simulink model "data_inspector_Baleka"  (R2024a)
settings: Solver=ode45  StartTime=0.0  StopTime=Sim.time  MaxStep=0.00001  RelTol=1e-12  AbsTol=1e-12
settings Model: Creator=heath  LastModifiedBy=Gavin

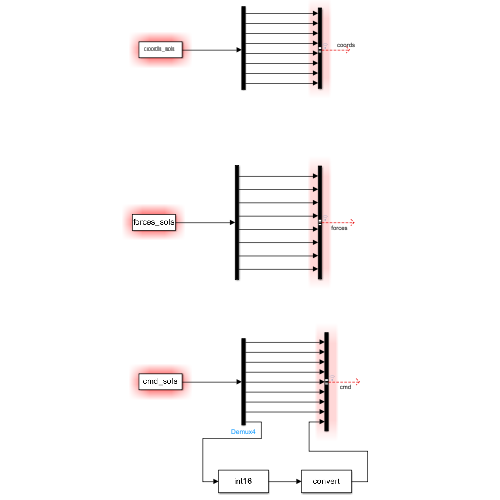
[thumbnail: Simulink's stored preview of the top-level diagram]
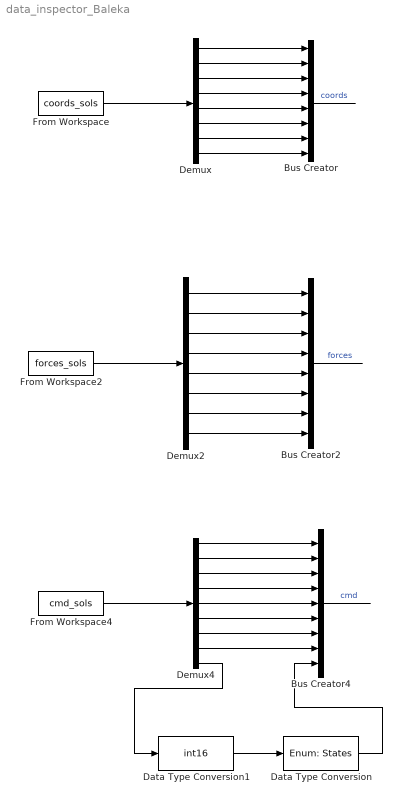
== system data_inspector_Baleka ==
  Bus Creator : BusCreator  Inputs=8  OutDataTypeStr=Bus: Coordinate
      settings: InheritFromInputs=off
  Bus Creator2 : BusCreator  Inputs=8  OutDataTypeStr=Bus: Forces
      settings: InheritFromInputs=off
  Bus Creator4 : BusCreator  Inputs=9  OutDataTypeStr=Bus: Cmd
      settings: InheritFromInputs=off
  Data Type Conversion : DataTypeConversion  OutDataTypeStr=Enum: States  SaturateOnIntegerOverflow=off  RndMeth=Floor
  Data Type Conversion1 : DataTypeConversion  OutDataTypeStr=int16  SaturateOnIntegerOverflow=off  RndMeth=Floor
  Demux : Demux  Outputs=8
  Demux2 : Demux  Outputs=8
  Demux4 : Demux  Outputs=9
  From Workspace : FromWorkspace  VariableName=coords_sols
  From Workspace2 : FromWorkspace  VariableName=forces_sols
  From Workspace4 : FromWorkspace  VariableName=cmd_sols
  wires:
  From Workspace2/1 -> Demux2/1
  Bus Creator/1 -> ?  "coords"
  Demux/8 -> Bus Creator/8
  Demux/7 -> Bus Creator/7
  Demux/6 -> Bus Creator/6
  Demux/5 -> Bus Creator/5
  Demux/4 -> Bus Creator/4
  Demux/3 -> Bus Creator/3
  Demux/2 -> Bus Creator/2
  Demux/1 -> Bus Creator/1
  From Workspace/1 -> Demux/1
  Bus Creator2/1 -> ?  "forces"
  From Workspace4/1 -> Demux4/1
  Demux4/2 -> Bus Creator4/2
  Demux4/1 -> Bus Creator4/1
  Demux4/5 -> Bus Creator4/5
  Demux4/3 -> Bus Creator4/3
  Demux4/4 -> Bus Creator4/4
  Bus Creator4/1 -> ?  "cmd"
  Demux2/6 -> Bus Creator2/6
  Demux2/5 -> Bus Creator2/5
  Demux2/4 -> Bus Creator2/4
  Demux2/3 -> Bus Creator2/3
  Demux2/2 -> Bus Creator2/2
  Demux2/1 -> Bus Creator2/1
  Demux4/6 -> Bus Creator4/6
  Data Type Conversion/1 -> Bus Creator4/9
  Data Type Conversion1/1 -> Data Type Conversion/1
  Demux2/7 -> Bus Creator2/7
  Demux2/8 -> Bus Creator2/8
  Demux4/9 -> Data Type Conversion1/1
  Demux4/8 -> Bus Creator4/8
  Demux4/7 -> Bus Creator4/7
